simulink model "q5_CS_Assignment"  (R2021b)
settings: Solver=ode4  StartTime=0.0  StopTime=tstop  FixedStep=tstep  RelTol=1e-3
libraries: simulink x1
settings Model: Creator=shash  LastModifiedBy=shash
settings DataIOCC: ReturnWorkspaceOutputs=off

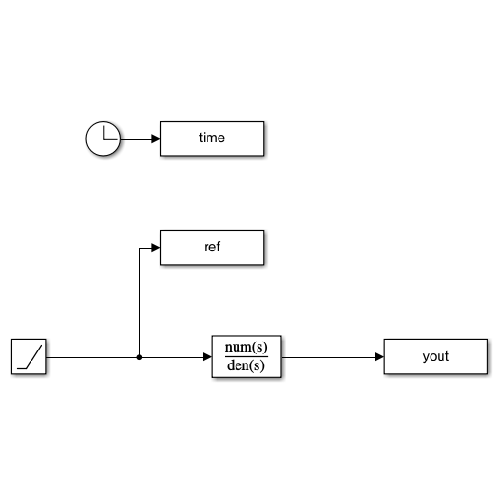
[thumbnail: Simulink's stored preview of the top-level diagram]
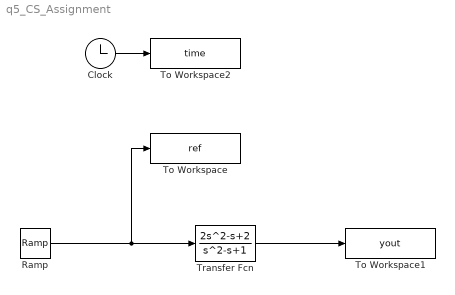
== system q5_CS_Assignment ==
  Clock : Clock
  Ramp : simulink/Sources/Ramp  slope=1  start=0  InitialOutput=0
  To Workspace : ToWorkspace  VariableName=ref  SampleTime=-1
  To Workspace1 : ToWorkspace  VariableName=yout  SampleTime=-1
  To Workspace2 : ToWorkspace  VariableName=time  SampleTime=-1
  Transfer Fcn : TransferFcn  Numerator=[2 -1 2]  Denominator=[1 -1 1]
  wires:
  Transfer Fcn/1 -> To Workspace1/1
  Ramp/1 -> To Workspace/1, Transfer Fcn/1
  Clock/1 -> To Workspace2/1
